simulink model "sim_trajectory_tracking"  (R2024b)
settings: Solver=VariableStepAuto  StartTime=0.0  StopTime=T_SIM  MaxStep=0.001  RelTol=0.04
values from neighbouring files (symbols this model uses):
  control_par = [k_1, k_2, k_3]    [regulation_script.m]    (also in traj_tracking_script.m = [k1, k2,b])
  controller_index = 2    [regulation_script.m]    (also in traj_tracking_script.m = 1)
  d = d_actual    (= 0.1694)    [regulation_script.m]    (also in traj_tracking_script.m = 0.165)
  d_actual = 0.1694    [regulation_script.m]    (also in traj_tracking_script.m = 0.165)
  omega_M = 10    [regulation_script.m]    (also in traj_tracking_script.m = 12)
  Q_INIT = [0;-2;pi/2+0.01]    [regulation_script.m]    (also in traj_tracking_script.m = [.2; 0.; pi/2])
  r = r_actual    (= 0.0302)    [regulation_script.m]    (also in traj_tracking_script.m = 0.03)
  r_actual = 0.0302    [regulation_script.m]    (also in traj_tracking_script.m = 0.03)
  T_trj = 18    [traj_tracking_script.m]
  trj_index = 1    [traj_tracking_script.m]
settings Model: Creator=alber  LastModifiedBy=loren
settings RTWCC: GPUComputeCapability=3.5

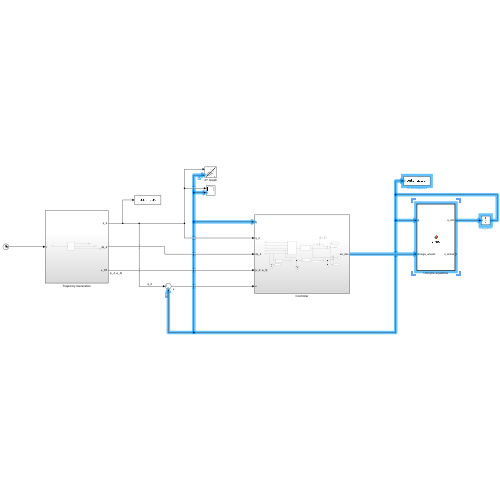
[thumbnail: Simulink's stored preview of the top-level diagram]
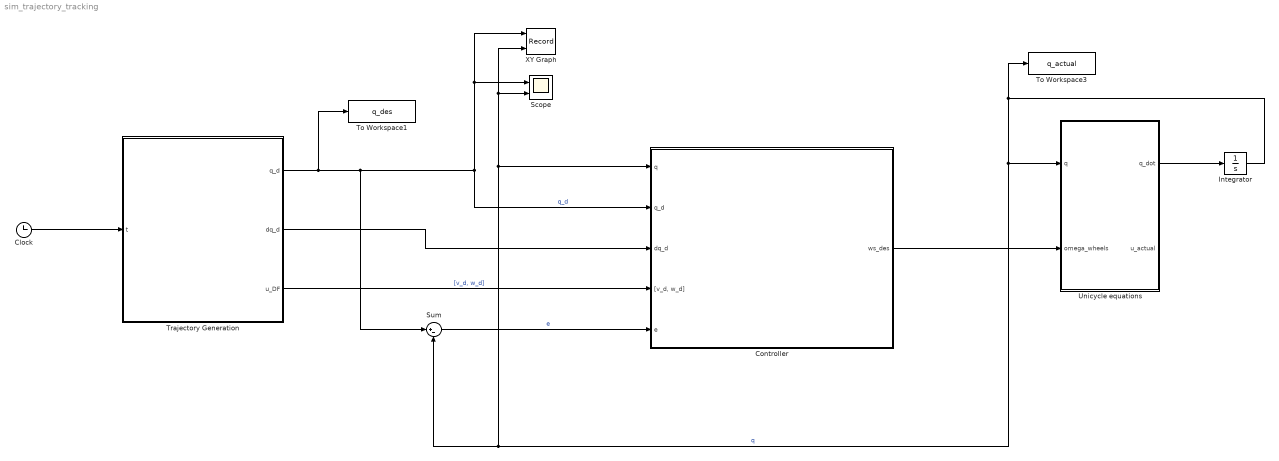
== system sim_trajectory_tracking ==
  Clock : Clock
  Controller : Subsystem
  Integrator : Integrator  InitialCondition=Q_INIT
  Scope : Scope  NumInputPorts=2
  Sum : Sum  Inputs=|+-
  To Workspace1 : ToWorkspace  VariableName=q_des  SaveFormat=Structure With Time  SampleTime=-1
  To Workspace3 : ToWorkspace  VariableName=q_actual  SaveFormat=Structure With Time  SampleTime=-1
  Trajectory Generation : Subsystem
  Unicycle equations : MATLAB Function  TreatAsAtomicUnit=on
  XY Graph : Record  FileSettingsInternal="{\"entries\":[{\"content\":{\"excelSettings\":{\"content\":{},\"type\":\"Streamout.ExcelSettings\"}},\"type\":\"Streamout.FileSettingStorage\",\"uuid\":\"\"}],\"packageUris\":[\"http:\\/\\/schema.mathworks.com\\/mf0\\/streamout_blocks\\/R2020a\"],\"version\":\"1.0\"}"  Layout=[1 1]  SignalsInternal="{\"entries\":[{\"content\":{\"signals\":[{\"content\":{\"blockPath\":[],\"dimensions\":[3,1],\"domain\":\"\",\"hasChildren\":true,\"lineColor\":\"#b746ff\",\"lineWidth\":2,\"port\":1,\"signalID\":1,\"signalName\":\"q_d\"},\"type\":\"RecordBlkView.Signal\",\"uuid\":\"\"},{\"content\":{\"blockPath\":[],\"channel\":[1,1],\"dimensions\":[3,1],\"domain\":\"\",\"lineColor\":\"#0072bd\",\"parentID\":1,\"port\":1,\"signalID\":2,\"signalName\":\"q_d\"},\"type\":\"RecordBlkView.Signal\",\"uuid\":\"\"},{\"content\":{\"blockPath\":[],\"channel\":[2,1],\"dimensions\":[3,1],\"domain\":\"\",\"lineColor\":\"#0072bd\",\"parentID\":1,\"plots\":[ 1 ],\"port\":1,\"signalID\":3,\"signalName\":\"q_d\"},\"type\":\"RecordBlkView.Signal\",\"uuid\":\"\"},{\"content\":{\"blockPath\":[],\"channel\":[3,1],\"dimensions\":[3,1],\"domain\":\"\",\"lineColor\":\"#139fff\",\"parentID\":1,\"port\":1,\"signalID\":4,\"signalName\":\"q_d\"},\"type\":\"RecordBlkView.Signal\",\"uuid\":\"\"},{\"content\":{\"blockPath\":[],\"dimensions\":[3,1],\"domain\":\"\",\"hasChildren\":true,\"lineColor\":\"#ff13a6\",\"lineWidth\":2,\"port\":2,\"signalID\":5,\"signalName\":\"q\"},\"type\":\"RecordBlkView.Signal\",\"uuid\":\"\"},{\"content\":{\"blockPath\":[],\"channel\":[1,1],\"dimensions\":[3,1],\"domain\":\"\",\"lineColor\":\"#000000\",\"lineStyle\":\"DASH_DOT\",\"parentID\":5,\"plots\":[ 1 ],\"port\":2,\"signalID\":6,\"signalName\":\"q\"},\"type\":\"RecordBlkView.Signal\",\"uuid\":\"\"},{\"content\":{\"blockPath\":[],\"channel\":[2,1],\"dimensions\":[3,1],\"domain\":\"\",\"lineColor\":\"#000000\",\"lineStyle\":\"DASH_DOT\",\"parentID\":5,\"plots\":[ 1 ],\"port\":2,\"signalID\":7,\"signalName\":\"q\"},\"type\":\"RecordBlkView.Signal\",\"uuid\":\"\"},{\"content\":{\"blockPath\":[],\"channel\":[3,1],\"dimensions\":[3,1],\"domain\":\"\",\"lineColor\":\"#b746ff\",\"parentID\":5,\"port\":2,\"signalID\":8,\"signalName\":\"q\"},\"type\":\"RecordBlkView.Signal\",\"uuid\":\"\"}]},\"type\":\"RecordBlkView.InputSignals\",\"uuid\":\"\"}],\"packageUris\":[\"http:\\/\\/schema.mathworks.com\\/mf0\\/streamout_blocks\\/R2020a\"],\"version\":\"1.0\"}"  VisualizationBindings="{\"xyplotplugin\":{\"info\":[{\"series\":[{\"bindingParametersList\":[{\"parameter\":\"Y-Axis\",\"signalID\":3,\"signalName\":\"q_d(2,1)\"}],\"seriesID\":0},{\"bindingParametersList\":[{\"parameter\":\"X-Axis\",\"signalID\":6,\"signalName\":\"q(1,1)\"},{\"parameter\":\"Y-Axis\",\"signalID\":7,\"signalName\":\"q(2,1)\"}],\"seriesID\":1}],\"subplotID\":1}]}}"  CompatibilityTag=XY
  wires:
  Integrator/1 -> To Workspace3/1, XY Graph/2, Scope/2, Controller/1(q), Sum/2, Unicycle equations/1(q)  "q"
  Unicycle equations/1(q_dot) -> Integrator/1
  Trajectory Generation/1(q_d) -> To Workspace1/1, Sum/1, Controller/2(q_d), XY Graph/1, Scope/1  "q_d"
  Clock/1 -> Trajectory Generation/1(t)
  Trajectory Generation/2(dq_d) -> Controller/3(dq_d)
  Trajectory Generation/3(u_DF) -> Controller/4("[v_d, w_d]")  "[v_d, w_d]"
  Sum/1 -> Controller/5(e)  "e"
  Controller/1(ws_des) -> Unicycle equations/2(omega_wheels)

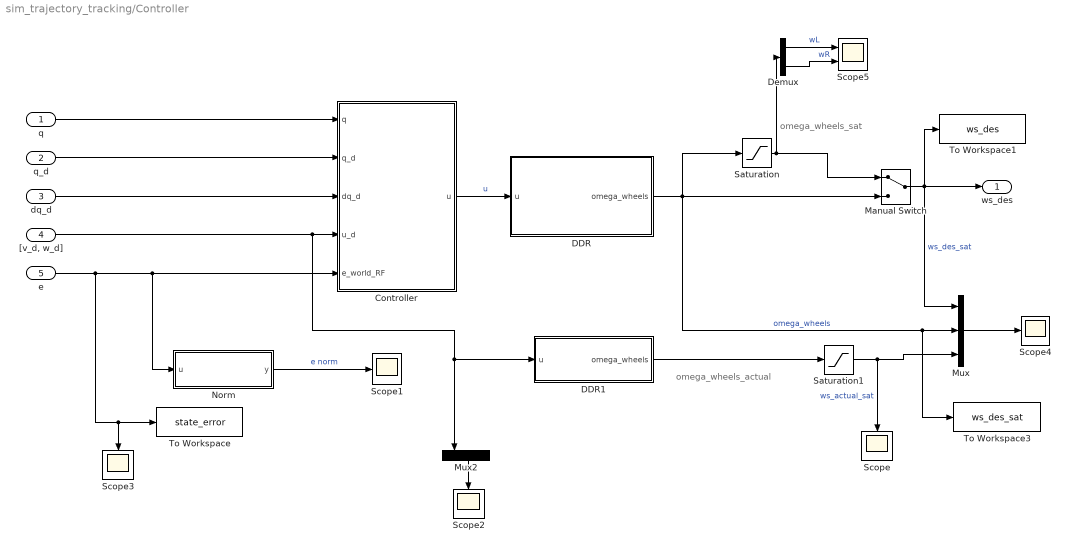
== system sim_trajectory_tracking/Controller ==
  note: omega_wheels_actual
  note: omega_wheels_sat
  q : Inport
  q_d : Inport  Port=2
  dq_d : Inport  Port=3
  "[v_d, w_d]" : Inport  Port=4
  e : Inport  Port=5
  Controller : MATLAB Function  TreatAsAtomicUnit=on
  DDR : MATLAB Function  TreatAsAtomicUnit=on
  DDR1 : MATLAB Function  TreatAsAtomicUnit=on
  Demux : Demux  Outputs=2
  Manual Switch : ManualSwitch
  Mux : Mux  Inputs=3
  Mux2 : Mux  Inputs=2
  Norm : MATLAB Function  TreatAsAtomicUnit=on
  Saturation : Saturate  UpperLimit=omega_M  LowerLimit=-omega_M
  Saturation1 : Saturate  UpperLimit=omega_M  LowerLimit=-omega_M
  Scope{,1..4} (5 alike) : Scope
  Scope5 : Scope  NumInputPorts=2
  To Workspace : ToWorkspace  VariableName=state_error  SaveFormat=Structure With Time  SampleTime=-1
  To Workspace1 : ToWorkspace  VariableName=ws_des  SaveFormat=Structure With Time  SampleTime=-1
  To Workspace3 : ToWorkspace  VariableName=ws_des_sat  SaveFormat=Structure With Time  SampleTime=-1
  ws_des : Outport
  wires:
  "[v_d, w_d]"/1 -> Mux2/1, DDR1/1(u), Controller/4(u_d)
  Mux2/1 -> Scope2/1
  Saturation1/1 -> Scope/1, Mux/3  "ws_actual_sat"
  q/1 -> Controller/1(q)
  e/1 -> Controller/5(e_world_RF), Norm/1(u), Scope3/1, To Workspace/1
  Controller/1(u) -> DDR/1(u)  "u"
  DDR1/1(omega_wheels) -> Saturation1/1
  DDR/1(omega_wheels) -> To Workspace3/1, Mux/2, Manual Switch/2, Saturation/1  "omega_wheels"
  Norm/1(y) -> Scope1/1  "e norm"
  q_d/1 -> Controller/2(q_d)
  dq_d/1 -> Controller/3(dq_d)
  Manual Switch/1 -> To Workspace1/1, Mux/1, ws_des/1  "ws_des_sat"
  Saturation/1 -> Demux/1, Manual Switch/1
  Mux/1 -> Scope4/1
  Demux/1 -> Scope5/1  "wL"
  Demux/2 -> Scope5/2  "wR"

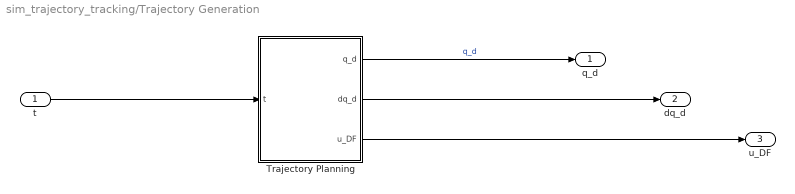
== system sim_trajectory_tracking/Trajectory Generation ==
  t : Inport
  Trajectory Planning : MATLAB Function  TreatAsAtomicUnit=on
  q_d : Outport
  dq_d : Outport  Port=2
  u_DF : Outport  Port=3
  wires:
  Trajectory Planning/1(q_d) -> q_d/1  "q_d"
  Trajectory Planning/2(dq_d) -> dq_d/1
  Trajectory Planning/3(u_DF) -> u_DF/1
  t/1 -> Trajectory Planning/1(t)

== matlab function sim_trajectory_tracking/Controller/Norm ==
  data: u input; y output
function y = fcn(u)

y = sqrt(sum(u(1:2).^2));

== matlab function sim_trajectory_tracking/Unicycle equations ==
  data: q input; omega_wheels input; q_dot output; r_actual parameter; d_actual parameter; u_actual output
function [q_dot, u_actual] = q_dot(q, omega_wheels, r_actual, d_actual)
    
    u_actual = [r_actual/2, r_actual/2;-r_actual/d_actual, r_actual/d_actual]*omega_wheels;
    
    theta = q(3);

    q_dot = [[cos(theta), 0];[sin(theta), 0];[0,1]] * u_actual;

== matlab function sim_trajectory_tracking/Trajectory Generation/Trajectory Planning ==
  data: t input; q_d output; dq_d output; u_DF output; trj_index parameter; T_trj parameter
function [q_d, dq_d, u_DF] = get_trj(t, trj_index, T_trj)
if trj_index == 1
    % line
    vel = 1/T_trj;
    q_d = [0; vel*t; pi/2];
    dq_d = [0; vel; 0];
    u_DF = [vel; 0];
elseif trj_index == 2
    % circle
    r = 0.5;
    omega = 2*pi/T_trj;
    theta_prime = omega*t;
    q_d = [r*cos(theta_prime); r*sin(theta_prime); theta_prime + pi/2];
    dq_d = [-omega*r*sin(theta_prime); omega*r*cos(theta_prime); omega];
    u_DF = [omega*r; omega];
elseif trj_index == 3
    %  square
    T_cycle = mod(t, T_trj);
    side_length = 1;
    vel = side_length/(T_trj/4);
    if T_cycle<=T_trj/4
        t_side = T_cycle;
        q_d = [0;  t_side*vel; pi/2];
        dq_d = [0;vel;0];
        u_DF = [vel; 0];
    elseif T_cycle <=T_trj/2
        t_side = T_cycle - T_trj/4;
        q_d = [-vel*t_side; side_length ;pi];
        dq_d = [-vel;0;0];
        u_DF = [vel;0];
    elseif T_cycle <= 3*T_trj/4
        t_side = T_cycle - T_trj/2;
        q_d = [-side_length; side_length-vel*t_side; -pi/2];
        dq_d = [0;-vel;0];
        u_DF = [vel;0];
    else
        t_side = T_cycle - 3*T_trj/4;
        q_d = [-side_length + vel*t_side; 0; 0];
        dq_d = [vel;0;0];
        u_DF = [vel;0];
    end
elseif trj_index == 4
    % 8-shape
    R = 0.4;
    omega = 2*pi/T_trj;
    x_d = R*sin(2*omega*t);
    dx_d = R*2*omega*cos(2*omega*t);
    ddx_d = -R*4*omega.^2*sin(2*omega*t);
    y_d = R*sin(omega*t);
    dy_d = R*omega*cos(omega*t);
    ddy_d = -R*omega.^2*sin(omega*t);
    theta_d = atan2(dy_d, dx_d);
    dtheta_d = (dx_d*ddy_d -  dy_d*ddx_d)/(dx_d.^2+dy_d.^2);
    q_d = [x_d;y_d;theta_d];
    dq_d = [dx_d;dy_d;dtheta_d];
    u_DF = [sqrt(dx_d.^2 + dy_d.^2);dtheta_d];


elseif trj_index == 5
    % S cartesian traj
    
    %% --- Parametri traiettoria
    Ta = 1;
    Tc = 10;
    qi = [-0.5; -0.5; pi/2];
    qf = [ 0.5;  0.5; pi/2];
    ki = 4;
    kf = 4;
    
    %% --- Time Law Trapezoidale (scalare in t) ---
    vc = 1 / (Ta + Tc);
    a  = vc / Ta;
    T_end = 2*Ta + Tc;
    
    if t < Ta
        % Fase 1: accelerazione
        s_dot = a * t;
        s     = 0.5 * a * t^2;
    elseif t < (Ta + Tc)
        % Fase 2: velocità costante
        s_dot = vc;
        s     = 0.5 * a * Ta^2 + vc * (t - Ta);
    elseif t < T_end
        % Fase 3: decelerazione
        dt3   = t - Ta - Tc;
        s_dot = vc - a * dt3;
        s     = 0.5*a*Ta^2 + vc*Tc + vc*dt3 - 0.5*a*dt3^2;
    else
        % Fase 4: fine traiettoria
        s_dot = 0;
        s     = 1;
    end
    
    %% --- Polinomi Cubici ---
    xi = qi(1); yi = qi(2); thetai = qi(3);
    xf = qf(1); yf = qf(2); thetaf = qf(3);
    
    coeff_a = [xf,  xi,  kf*cos(thetaf) - 3*xf,  ki*cos(thetai) + 3*xi];
    coeff_b = [yf,  yi,  kf*sin(thetaf) - 3*yf,  ki*sin(thetai) + 3*yi];
    
    % Posizione geometrica
    x_s = coeff_a(1)*s^3 - coeff_a(2)*(s^3-3*s^2+3*s-1) ...
        + coeff_a(3)*(s^3-s^2) + coeff_a(4)*(s^3-2*s^2+s);
    y_s = coeff_b(1)*s^3 - coeff_b(2)*(s^3-3*s^2+3*s-1) ...
        + coeff_b(3)*(s^3-s^2) + coeff_b(4)*(s^3-2*s^2+s);
    
    % Prima derivata rispetto a s
    x_ds = 3*coeff_a(1)*s^2 - coeff_a(2)*(3*s^2-6*s+3) ...
         + coeff_a(3)*(3*s^2-2*s) + coeff_a(4)*(3*s^2-4*s+1);
    y_ds = 3*coeff_b(1)*s^2 - coeff_b(2)*(3*s^2-6*s+3) ...
         + coeff_b(3)*(3*s^2-2*s) + coeff_b(4)*(3*s^2-4*s+1);
    
    % Seconda derivata rispetto a s
    x_dds = 6*coeff_a(1)*s - coeff_a(2)*(6*s-6) + coeff_a(3)*(6*s-2) + coeff_a(4)*(6*s-4);
    y_dds = 6*coeff_b(1)*s - coeff_b(2)*(6*s-6) + coeff_b(3)*(6*s-2) + coeff_b(4)*(6*s-4);
    
    %% --- Input geometrici ---
    v_tilde     = sqrt(x_ds^2 + y_ds^2);
    omega_tilde = (x_ds * y_dds - y_ds * x_dds) / (x_ds^2 + y_ds^2);
    
    %% --- Input reali (feedforward) ---
    v = v_tilde * s_dot;
    w = omega_tilde * s_dot;

    u_DF = [v;w];
    
    %% --- Stato desiderato q_d = [x; y; theta] ---
    theta_d = atan2(y_ds, x_ds);   % orientamento tangente alla curva
    q_d  = [x_s; y_s; theta_d];
    
    %% --- Velocità desiderata dq_d = [dx; dy; dtheta] ---
    % Per un unicycle: dx = v*cos(theta), dy = v*sin(theta), dtheta = w
    dq_d = [v * cos(theta_d);
            v * sin(theta_d);
            w];
else
    q_d = [0;0;0];
    dq_d = [0;0;0];
    u_DF = [0;0];
end

== matlab function sim_trajectory_tracking/Controller/Controller ==
  data: q input; q_d input; dq_d input; u_d input; u output; e_world_RF input; controller_index parameter; control_par parameter
function u = fcn(q, q_d, dq_d, u_d, e_world_RF, controller_index, control_par)

    % LINREAR controller
    if controller_index == 1
                
        vd = u_d(1); wd = u_d(2);

        % derive control matrix K
        K = linear_gains(control_par, vd, wd);
        k1 = K(1); k2 = K(2); k3 = K(3);

        % rotation of the error
        e_body = error_rotation(e_world_RF, q);
        e1 = e_body(1); e2 = e_body(2); e3 = e_body(3); 
    
        % Linear Contrl Law
        % Define u_aux_1, u_aux_2 auxiliar inputs
        u1_aux = -k1 * e1;
        u2_aux = -k2 * e2 - k3 * e3;
        
        % 3. Real model inputs    
        v = vd * cos(e3) - u1_aux;
        w = wd - u2_aux;
        
        % Saturation (if i want a saturation directly on v and w
        % v = max(min(v, 1.5), -1.5); 
        % w = max(min(w, 3.0), -3.0);
        
        u = [v; w];


    % --------------------------------------
    % NON LINEAR controller
    elseif controller_index == 2
        
        vd = u_d(1); wd = u_d(2);

        % derive control matrix K
        K = NL_gains(control_par, vd, wd);
        k1 = K(1); k2 = K(2); k3 = K(3); 

        % rotation of the error
        e_body = error_rotation(e_world_RF, q);
        e1 = e_body(1); e2 = e_body(2); e3 = e_body(3); 
    
        % NON-Linear Contrl Law
        
        % Singularity: sinc(e3) = sin(e3)/e3
        if abs(e3) < 1e-4
            sinc_e3 = 1;
        else
            sinc_e3 = sin(e3)/e3;
        end
        
        % Define u_aux_1, u_aux_2 auxiliar inputs
        u1_aux = -k1 * e1;
        u2_aux = -k2 * vd * sinc_e3 * e2 - k3 * e3;
       
        % Real model inputs
        v = vd * cos(e3) - u1_aux;
        w = wd - u2_aux;
        
        % Saturation  
        % v = max(min(v, 1.5), -1.5); 
        % w = max(min(w, 3.0), -3.0);
        
        u = [v; w];


    % --------------------------------------
    % FEEDBACK LINEARIZATION (OUTPUT ERROR FB)
    elseif controller_index == 3
    % here it is considered q the B_point_q, the same for q_d and the error

        theta = q(3);
        k1 = control_par(1); k2 = control_par(2); b = control_par(3);

        % build K matrix
        K = [k1 , 0 ; 0 , k2];

        % I just need the the first 2 components of the error (ep_x, ep_y)
        % in the world frame
        ep = [ e_world_RF(1) ; e_world_RF(2) ];
  
        % same for the pose
        pBd_dot = [ dq_d(1) ; dq_d(2) ];
        
        T_inv = [cos(theta),       sin(theta);
                 -(1/b) * sin(theta), (1/b) * cos(theta)];
    
        u = T_inv * (pBd_dot + K * ep);     % u = [v; w]

    else
        u = u_d;
    end
end

% ------------------------------------------------------------------

% LOCAL FUNCTIONS


function e_body = error_rotation(e_w, q)

    % Extracts the current robot orientation
    theta = q(3);
    
    % Normalize the orientation error (3rd component) to be within [-pi, pi]
    % This prevents the robot from making unnecessary 360-degree turns.
    e_theta = e_w(3);
    e_w(3) = atan2(sin(e_theta), cos(e_theta));
    
    % Rotation matrix transpose
    R_T = [ cos(theta), sin(theta), 0;
           -sin(theta), cos(theta), 0;
                0,          0,      1];
            
    % Compute error in Body Frame
    e_body = R_T * e_w;

end
    
function K = linear_gains(control_par, vd, wd)
    xi = control_par(1);
    a = control_par(2);

    k1 = 2 * xi * a; 
    k3 = k1;
    
    % if vd is zero the gain will be huge (controlled then by saturation)
    if abs(vd) < 1e-4
        if vd >= 0
            vd = 1e-4;
        else
            vd = -1e-4;
        end
    end
        
    k2 = (a^2 - wd^2)/vd;

    K = [k1; k2; k3];
end


function K = NL_gains(control_par, vd, wd)
    xi = control_par(1);
    b = control_par(2);

    k1 = 2 * xi * sqrt(b*vd + wd^2); 
    k3 = k1;
    k2 = b;

    K = [k1; k2; k3];
end

== matlab function sim_trajectory_tracking/Controller/DDR ==
  data: u input; omega_wheels output; r parameter; d parameter
function omega_wheels = kin2omegawheels(u, r, d)

omega_l = u(1)/r-d/(2*r)*u(2);
omega_r = u(1)/r+d/(2*r)*u(2);

omega_wheels = [omega_l;omega_r];

== matlab function sim_trajectory_tracking/Controller/DDR1 ==
  data: u input; omega_wheels output; r_actual parameter; d_actual parameter
function omega_wheels = kin2omegawheels(u, r_actual, d_actual)
omega_l = u(1)/r_actual-d_actual/(2*r_actual)*u(2);
omega_r = u(1)/r_actual+d_actual/(2*r_actual)*u(2);
omega_wheels = [omega_l;omega_r];
